simulink model "NCSEx3_sim"  (R2024b)
settings: Solver=VariableStepAuto  StartTime=0.0  StopTime=NCS.simTime  FixedStep=Td  RelTol=1e-3
InitFcn:
  | set_param(gcs, 'SimulationCommand', 'update')
values from neighbouring files (symbols this model uses):
  NCS = NcsStructureEx3(ncsPlant, 'simTime', simTime,                     'networkEffectsData', networkEffectsData,                     'controlParams', controlParams,                     'observerParams', observerParams)    [mainEx3.m]
undefined symbols (not defined in the file or in its folder): sfunchk
libraries: cstblocks x1, truetime x1
settings Model: Creator=jakob_ludwiger  LastModifiedBy=kala
settings SolverCC: AlgebraicLoopSolver=TrustRegion
settings DataIOCC: ReturnWorkspaceOutputs=off
settings DebuggingCC: UnconnectedInputMsg=warning  UnconnectedOutputMsg=warning  UnconnectedLineMsg=warning  ArithmeticOperatorsInVariantConditions=warning
settings ModelReferenceCC: EnableRefExpFcnMdlSchedulingChecks=on
settings SFSimCC: SimUseLocalCustomCode=off  CustomCodeUndefinedFunction=UseInterfaceOnly
settings RTWCC: RTWUseLocalCustomCode=off  GPUComputeCapability=3.5  DLArmComputeVersion=19.05
settings CodeAppCC: StateflowObjectComments=on

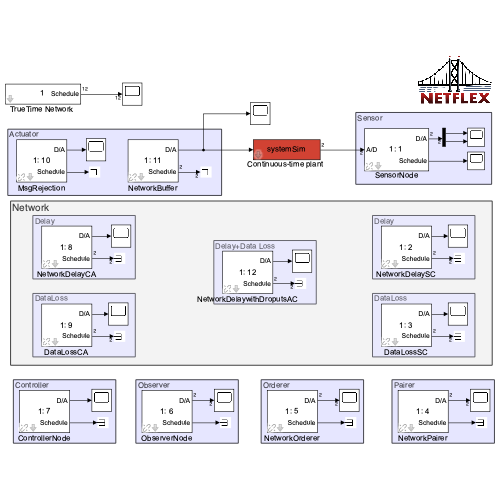
[thumbnail: Simulink's stored preview of the top-level diagram]
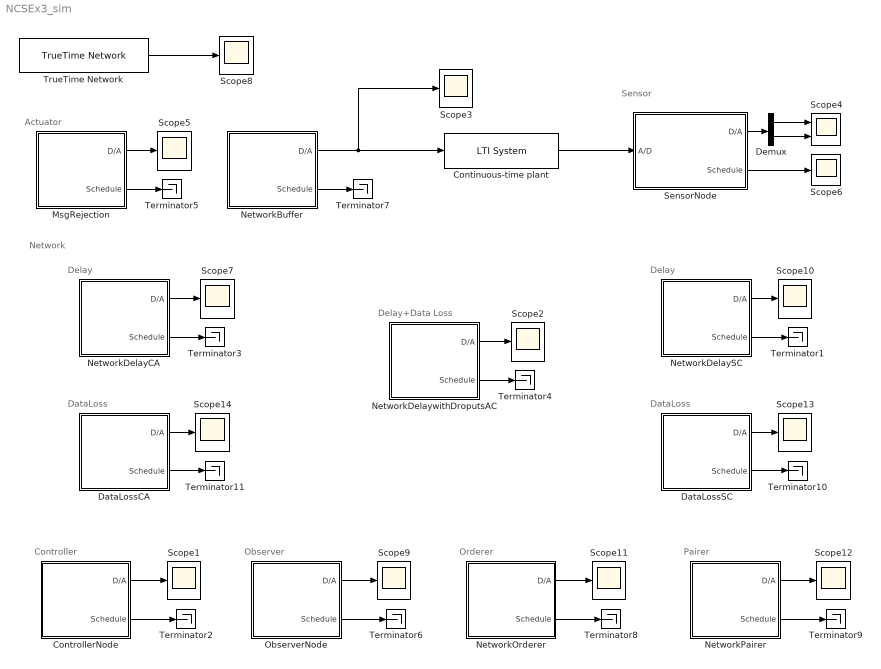
== system NCSEx3_sim ==
  note: Network
  note: Sensor
  note: Delay
  note: Delay
  note: Actuator
  note: Controller
  note: Delay+Data Loss
  note: Observer
  note: Orderer
  note: Pairer
  note: DataLoss
  note: DataLoss
  "Continuous-time plant " : cstblocks/LTI System  sys=systemSim  IC=initialState  PadeOrder=0
  ControllerNode : Subsystem  AncestorBlock=truetime/TrueTime Kernel  InitFcn=sfunchk(get_param(gcb,'sfun'));  mask{nodeObj=NCS.nodeMap('ControllerNode'), sfun=initFctWrapper, ntriggers=0, trigtype=falling, clockoffsetdrift=[0 0], schedoutput=on, battery=off, poweroutput=off, label=1: 7}
      mask prompts: nodeObj "Node Object"; sfun "Name of init function (MEX or MATLAB):"; ntriggers "Number of external triggers:"; trigtype "Trigger type:"; clockoffsetdrift "Local clock offset and drift:"; schedoutput "Show Schedule output port"; battery "Show Energy supply input port"; poweroutput "Show Power consumption output port"
      mask init:
      | set_param(gcb,'sfun', nodeObj.initFunctionWrapper)
      | %set_param(gcb,'args', [3 2])
      | args = nodeObj;
      | ninputsoutputs = [nodeObj.nIn nodeObj.nOut];
      | nwnodenbr = nodeObj.nodeNr;
      | ttkernel_callback(gcb,{sfun,args,ninputsoutputs,ntriggers,trigtype,nwnodenbr,clockoffsetdrift,schedoutput,battery,poweroutput})
      settings: ErrorFcn=ttkernel_error
      mask TypeOptions trigtype: rising | falling | either
      mask Display: disp(get_param(gcb,'label'))
  DataLossCA : Subsystem  AncestorBlock=truetime/TrueTime Kernel  InitFcn=sfunchk(get_param(gcb,'sfun'));  mask{nodeObj=NCS.nodeMap('NetworkDropoutCA'), sfun=initFctWrapper, ntriggers=0, trigtype=falling, clockoffsetdrift=[0 0], schedoutput=on, battery=off, poweroutput=off, label=1: 9}
      mask prompts: nodeObj "Node Object"; sfun "Name of init function (MEX or MATLAB):"; ntriggers "Number of external triggers:"; trigtype "Trigger type:"; clockoffsetdrift "Local clock offset and drift:"; schedoutput "Show Schedule output port"; battery "Show Energy supply input port"; poweroutput "Show Power consumption output port"
      mask init: same as NCSEx3_sim/ControllerNode
      settings: ErrorFcn=ttkernel_error
      mask TypeOptions trigtype: rising | falling | either
      mask Display: disp(get_param(gcb,'label'))
  DataLossSC : Subsystem  AncestorBlock=truetime/TrueTime Kernel  InitFcn=sfunchk(get_param(gcb,'sfun'));  mask{nodeObj=NCS.nodeMap('NetworkDropoutSC'), sfun=initFctWrapper, ntriggers=0, trigtype=falling, clockoffsetdrift=[0 0], schedoutput=on, battery=off, poweroutput=off, label=1: 3}
      mask prompts: nodeObj "Node Object"; sfun "Name of init function (MEX or MATLAB):"; ntriggers "Number of external triggers:"; trigtype "Trigger type:"; clockoffsetdrift "Local clock offset and drift:"; schedoutput "Show Schedule output port"; battery "Show Energy supply input port"; poweroutput "Show Power consumption output port"
      mask init: same as NCSEx3_sim/ControllerNode
      settings: ErrorFcn=ttkernel_error
      mask TypeOptions trigtype: rising | falling | either
      mask Display: disp(get_param(gcb,'label'))
  Demux : Demux  Outputs=2
  MsgRejection : Subsystem  AncestorBlock=truetime/TrueTime Kernel  InitFcn=sfunchk(get_param(gcb,'sfun'));  mask{nodeObj=NCS.nodeMap('MsgRejection'), sfun=initFctWrapper, ntriggers=0, trigtype=falling, clockoffsetdrift=[0 0], schedoutput=on, battery=off, poweroutput=off, label=1: 10}
      mask prompts: nodeObj "Node Object"; sfun "Name of init function (MEX or MATLAB):"; ntriggers "Number of external triggers:"; trigtype "Trigger type:"; clockoffsetdrift "Local clock offset and drift:"; schedoutput "Show Schedule output port"; battery "Show Energy supply input port"; poweroutput "Show Power consumption output port"
      mask init: same as NCSEx3_sim/ControllerNode
      settings: ErrorFcn=ttkernel_error
      mask TypeOptions trigtype: rising | falling | either
      mask Display: disp(get_param(gcb,'label'))
  NetworkBuffer : Subsystem  AncestorBlock=truetime/TrueTime Kernel  InitFcn=sfunchk(get_param(gcb,'sfun'));  mask{nodeObj=NCS.nodeMap('NetworkBuffer'), sfun=initFctWrapper, ntriggers=0, trigtype=falling, clockoffsetdrift=[0 0], schedoutput=on, battery=off, poweroutput=off, label=1: 11}
      mask prompts: nodeObj "Node Object"; sfun "Name of init function (MEX or MATLAB):"; ntriggers "Number of external triggers:"; trigtype "Trigger type:"; clockoffsetdrift "Local clock offset and drift:"; schedoutput "Show Schedule output port"; battery "Show Energy supply input port"; poweroutput "Show Power consumption output port"
      mask init: same as NCSEx3_sim/ControllerNode
      settings: ErrorFcn=ttkernel_error
      mask TypeOptions trigtype: rising | falling | either
      mask Display: disp(get_param(gcb,'label'))
  NetworkDelayCA : Subsystem  AncestorBlock=truetime/TrueTime Kernel  InitFcn=sfunchk(get_param(gcb,'sfun'));  mask{nodeObj=NCS.nodeMap('NetworkDelayCA'), sfun=initFctWrapper, ntriggers=0, trigtype=falling, clockoffsetdrift=[0 0], schedoutput=on, battery=off, poweroutput=off, label=1: 8}
      mask prompts: nodeObj "Node Object"; sfun "Name of init function (MEX or MATLAB):"; ntriggers "Number of external triggers:"; trigtype "Trigger type:"; clockoffsetdrift "Local clock offset and drift:"; schedoutput "Show Schedule output port"; battery "Show Energy supply input port"; poweroutput "Show Power consumption output port"
      mask init: same as NCSEx3_sim/ControllerNode
      settings: ErrorFcn=ttkernel_error
      mask TypeOptions trigtype: rising | falling | either
      mask Display: disp(get_param(gcb,'label'))
  NetworkDelaySC : Subsystem  AncestorBlock=truetime/TrueTime Kernel  InitFcn=sfunchk(get_param(gcb,'sfun'));  mask{nodeObj=NCS.nodeMap('NetworkDelaySC'), sfun=initFctWrapper, ntriggers=0, trigtype=falling, clockoffsetdrift=[0 0], schedoutput=on, battery=off, poweroutput=off, label=1: 2}
      mask prompts: nodeObj "Node Object"; sfun "Name of init function (MEX or MATLAB):"; ntriggers "Number of external triggers:"; trigtype "Trigger type:"; clockoffsetdrift "Local clock offset and drift:"; schedoutput "Show Schedule output port"; battery "Show Energy supply input port"; poweroutput "Show Power consumption output port"
      mask init: same as NCSEx3_sim/ControllerNode
      settings: ErrorFcn=ttkernel_error
      mask TypeOptions trigtype: rising | falling | either
      mask Display: disp(get_param(gcb,'label'))
  NetworkDelaywithDroputsAC : Subsystem  AncestorBlock=truetime/TrueTime Kernel  InitFcn=sfunchk(get_param(gcb,'sfun'));  mask{nodeObj=NCS.nodeMap('NetworkDelayWithDropoutsAC'), sfun=initFctWrapper, ntriggers=0, trigtype=falling, clockoffsetdrift=[0 0], schedoutput=on, battery=off, poweroutput=off, label=1: 12}
      mask prompts: nodeObj "Node Object"; sfun "Name of init function (MEX or MATLAB):"; ntriggers "Number of external triggers:"; trigtype "Trigger type:"; clockoffsetdrift "Local clock offset and drift:"; schedoutput "Show Schedule output port"; battery "Show Energy supply input port"; poweroutput "Show Power consumption output port"
      mask init: same as NCSEx3_sim/ControllerNode
      settings: ErrorFcn=ttkernel_error
      mask TypeOptions trigtype: rising | falling | either
      mask Display: disp(get_param(gcb,'label'))
  NetworkOrderer : Subsystem  AncestorBlock=truetime/TrueTime Kernel  InitFcn=sfunchk(get_param(gcb,'sfun'));  mask{nodeObj=NCS.nodeMap('NetworkOrderer'), sfun=initFctWrapper, ntriggers=0, trigtype=falling, clockoffsetdrift=[0 0], schedoutput=on, battery=off, poweroutput=off, label=1: 5}
      mask prompts: nodeObj "Node Object"; sfun "Name of init function (MEX or MATLAB):"; ntriggers "Number of external triggers:"; trigtype "Trigger type:"; clockoffsetdrift "Local clock offset and drift:"; schedoutput "Show Schedule output port"; battery "Show Energy supply input port"; poweroutput "Show Power consumption output port"
      mask init: same as NCSEx3_sim/ControllerNode
      settings: ErrorFcn=ttkernel_error
      mask TypeOptions trigtype: rising | falling | either
      mask Display: disp(get_param(gcb,'label'))
  NetworkPairer : Subsystem  AncestorBlock=truetime/TrueTime Kernel  InitFcn=sfunchk(get_param(gcb,'sfun'));  mask{nodeObj=NCS.nodeMap('NetworkPairer'), sfun=initFctWrapper, ntriggers=0, trigtype=falling, clockoffsetdrift=[0 0], schedoutput=on, battery=off, poweroutput=off, label=1: 4}
      mask prompts: nodeObj "Node Object"; sfun "Name of init function (MEX or MATLAB):"; ntriggers "Number of external triggers:"; trigtype "Trigger type:"; clockoffsetdrift "Local clock offset and drift:"; schedoutput "Show Schedule output port"; battery "Show Energy supply input port"; poweroutput "Show Power consumption output port"
      mask init: same as NCSEx3_sim/ControllerNode
      settings: ErrorFcn=ttkernel_error
      mask TypeOptions trigtype: rising | falling | either
      mask Display: disp(get_param(gcb,'label'))
  ObserverNode : Subsystem  AncestorBlock=truetime/TrueTime Kernel  InitFcn=sfunchk(get_param(gcb,'sfun'));  mask{nodeObj=NCS.nodeMap('ObserverNode'), sfun=initFctWrapper, ntriggers=0, trigtype=falling, clockoffsetdrift=[0 0], schedoutput=on, battery=off, poweroutput=off, label=1: 6}
      mask prompts: nodeObj "Node Object"; sfun "Name of init function (MEX or MATLAB):"; ntriggers "Number of external triggers:"; trigtype "Trigger type:"; clockoffsetdrift "Local clock offset and drift:"; schedoutput "Show Schedule output port"; battery "Show Energy supply input port"; poweroutput "Show Power consumption output port"
      mask init: same as NCSEx3_sim/ControllerNode
      settings: ErrorFcn=ttkernel_error
      mask TypeOptions trigtype: rising | falling | either
      mask Display: disp(get_param(gcb,'label'))
  Scope{1..3,5..14} (13 alike) : Scope
  Scope4 : Scope  NumInputPorts=2
  SensorNode : Subsystem  AncestorBlock=truetime/TrueTime Kernel  InitFcn=sfunchk(get_param(gcb,'sfun'));  mask{nodeObj=NCS.nodeMap('SensorNode'), sfun=initFctWrapper, ntriggers=0, trigtype=falling, clockoffsetdrift=[0 0], schedoutput=on, battery=off, poweroutput=off, label=1: 1}
      mask prompts: nodeObj "Node Object"; sfun "Name of init function (MEX or MATLAB):"; ntriggers "Number of external triggers:"; trigtype "Trigger type:"; clockoffsetdrift "Local clock offset and drift:"; schedoutput "Show Schedule output port"; battery "Show Energy supply input port"; poweroutput "Show Power consumption output port"
      mask init: same as NCSEx3_sim/ControllerNode
      settings: ErrorFcn=ttkernel_error
      mask TypeOptions trigtype: rising | falling | either
      mask Display: disp(get_param(gcb,'label'))
  Terminator{1..11} (11 alike) : Terminator
  "TrueTime Network " : truetime/TrueTime Network  nwtype=CSMA/CD (Ethernet)  nwnbr=1  nnodes=NCS.getMaxNodeNr  rate=1e8  minsize=200  lossprob=0  seed=0  bandwidths=[0.5 0.5]  slotsize=512  schedule=[1 1 2]  memsize=80000  buftype=Common buffer  overflow=Retransmit  dynSchedule=0  miniSlotSize=0  NIT=0  QSortMode=FIFO  sync=0  irtSchedule=0  nrtLength=0  nodeGraph=0  scheduleoutput=on
  wires:
  SensorNode/2(Schedule) -> Scope6/1
  SensorNode/1(D/A) -> Demux/1
  "Continuous-time plant "/1 -> SensorNode/1(A/D)
  "TrueTime Network "/1 -> Scope8/1
  NetworkDelaySC/2(Schedule) -> Terminator1/1
  NetworkDelaySC/1(D/A) -> Scope10/1
  NetworkDelayCA/1(D/A) -> Scope7/1
  NetworkDelayCA/2(Schedule) -> Terminator3/1
  MsgRejection/2(Schedule) -> Terminator5/1
  MsgRejection/1(D/A) -> Scope5/1
  NetworkBuffer/2(Schedule) -> Terminator7/1
  ControllerNode/1(D/A) -> Scope1/1
  ControllerNode/2(Schedule) -> Terminator2/1
  NetworkBuffer/1(D/A) -> Scope3/1, "Continuous-time plant "/1
  NetworkDelaywithDroputsAC/2(Schedule) -> Terminator4/1
  NetworkDelaywithDroputsAC/1(D/A) -> Scope2/1
  ObserverNode/2(Schedule) -> Terminator6/1
  ObserverNode/1(D/A) -> Scope9/1
  NetworkOrderer/1(D/A) -> Scope11/1
  NetworkOrderer/2(Schedule) -> Terminator8/1
  NetworkPairer/2(Schedule) -> Terminator9/1
  NetworkPairer/1(D/A) -> Scope12/1
  Demux/1 -> Scope4/1
  Demux/2 -> Scope4/2
  DataLossSC/1(D/A) -> Scope13/1
  DataLossSC/2(Schedule) -> Terminator10/1
  DataLossCA/2(Schedule) -> Terminator11/1
  DataLossCA/1(D/A) -> Scope14/1

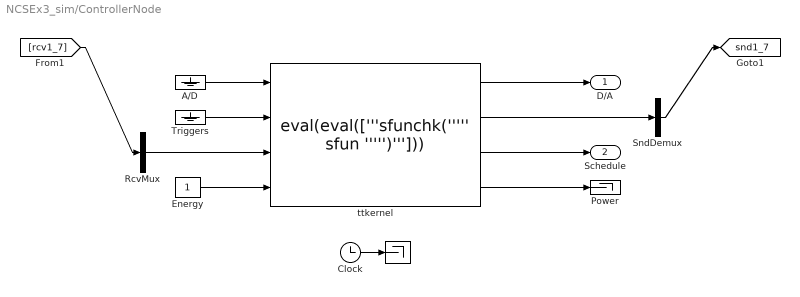
== system NCSEx3_sim/ControllerNode ==
  " " : Terminator
  A/D : Ground
  Clock : Clock
  Energy : Constant
  Power : Terminator
  RcvMux : Mux  Inputs=1
  SndDemux : Demux  Outputs=1
      settings: DisplayOption=none
  Triggers : Ground
  ttkernel : S-Function  FunctionName=eval(eval(['''sfunchk(''''' sfun ''''')''']))  Parameters=sfun, args, ninputsoutputs, ntriggers, trigtype, nwnodenbr, clockoffsetdrift  SFunctionDeploymentMode=off  EnableBusSupport=off
  D/A : Outport
  Schedule : Outport  Port=2
  tag scope: snd1_7=global
  wires:
  ttkernel/4 -> Power/1
  Energy/1 -> ttkernel/4
  A/D/1 -> ttkernel/1
  ttkernel/2 -> SndDemux/1
  ttkernel/1 -> D/A/1
  ttkernel/3 -> Schedule/1
  Triggers/1 -> ttkernel/2
  RcvMux/1 -> ttkernel/3
  Clock/1 -> " "/1
  [rcv1_7] -> RcvMux/1
  SndDemux/1 -> [snd1_7]

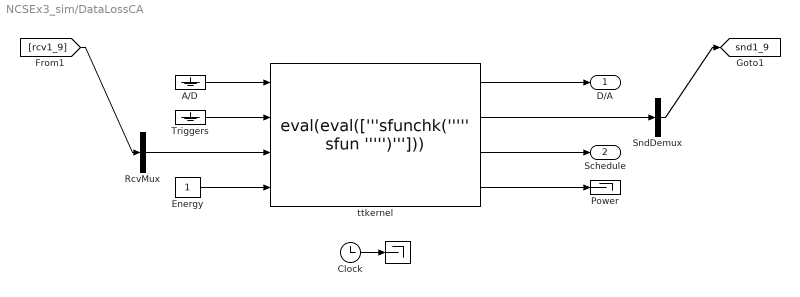
== system NCSEx3_sim/DataLossCA ==
  " " : Terminator
  A/D : Ground
  Clock : Clock
  Energy : Constant
  Power : Terminator
  RcvMux : Mux  Inputs=1
  SndDemux : Demux  Outputs=1
      settings: DisplayOption=none
  Triggers : Ground
  ttkernel : S-Function  FunctionName=eval(eval(['''sfunchk(''''' sfun ''''')''']))  Parameters=sfun, args, ninputsoutputs, ntriggers, trigtype, nwnodenbr, clockoffsetdrift  SFunctionDeploymentMode=off  EnableBusSupport=off
  D/A : Outport
  Schedule : Outport  Port=2
  tag scope: snd1_9=global
  wires:
  Clock/1 -> " "/1
  RcvMux/1 -> ttkernel/3
  Triggers/1 -> ttkernel/2
  ttkernel/3 -> Schedule/1
  ttkernel/1 -> D/A/1
  ttkernel/2 -> SndDemux/1
  A/D/1 -> ttkernel/1
  Energy/1 -> ttkernel/4
  ttkernel/4 -> Power/1
  [rcv1_9] -> RcvMux/1
  SndDemux/1 -> [snd1_9]

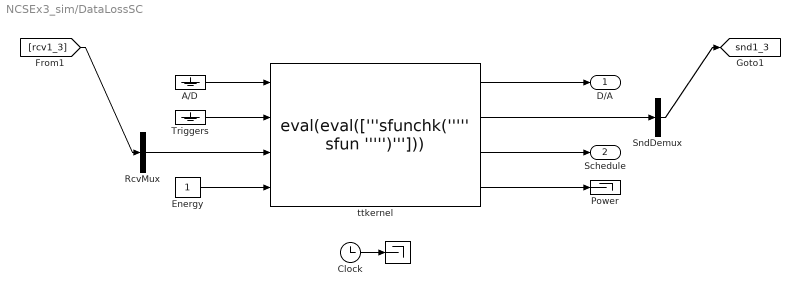
== system NCSEx3_sim/DataLossSC ==
  " " : Terminator
  A/D : Ground
  Clock : Clock
  Energy : Constant
  Power : Terminator
  RcvMux : Mux  Inputs=1
  SndDemux : Demux  Outputs=1
      settings: DisplayOption=none
  Triggers : Ground
  ttkernel : S-Function  FunctionName=eval(eval(['''sfunchk(''''' sfun ''''')''']))  Parameters=sfun, args, ninputsoutputs, ntriggers, trigtype, nwnodenbr, clockoffsetdrift  SFunctionDeploymentMode=off  EnableBusSupport=off
  D/A : Outport
  Schedule : Outport  Port=2
  tag scope: snd1_3=global
  wires:
  ttkernel/4 -> Power/1
  Energy/1 -> ttkernel/4
  A/D/1 -> ttkernel/1
  ttkernel/2 -> SndDemux/1
  ttkernel/1 -> D/A/1
  ttkernel/3 -> Schedule/1
  Triggers/1 -> ttkernel/2
  RcvMux/1 -> ttkernel/3
  Clock/1 -> " "/1
  [rcv1_3] -> RcvMux/1
  SndDemux/1 -> [snd1_3]

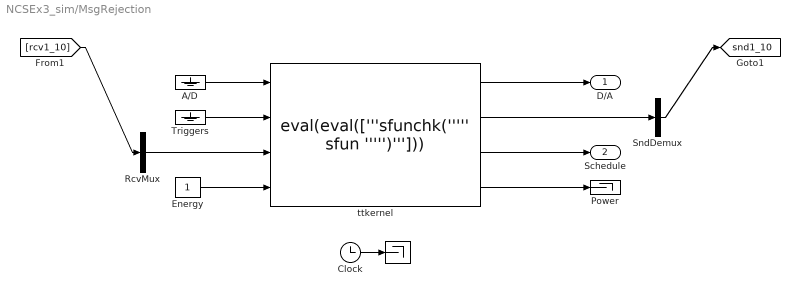
== system NCSEx3_sim/MsgRejection ==
  " " : Terminator
  A/D : Ground
  Clock : Clock
  Energy : Constant
  Power : Terminator
  RcvMux : Mux  Inputs=1
  SndDemux : Demux  Outputs=1
      settings: DisplayOption=none
  Triggers : Ground
  ttkernel : S-Function  FunctionName=eval(eval(['''sfunchk(''''' sfun ''''')''']))  Parameters=sfun, args, ninputsoutputs, ntriggers, trigtype, nwnodenbr, clockoffsetdrift  SFunctionDeploymentMode=off  EnableBusSupport=off
  D/A : Outport
  Schedule : Outport  Port=2
  tag scope: snd1_10=global
  wires:
  Clock/1 -> " "/1
  RcvMux/1 -> ttkernel/3
  Triggers/1 -> ttkernel/2
  ttkernel/3 -> Schedule/1
  ttkernel/1 -> D/A/1
  ttkernel/2 -> SndDemux/1
  A/D/1 -> ttkernel/1
  Energy/1 -> ttkernel/4
  ttkernel/4 -> Power/1
  [rcv1_10] -> RcvMux/1
  SndDemux/1 -> [snd1_10]

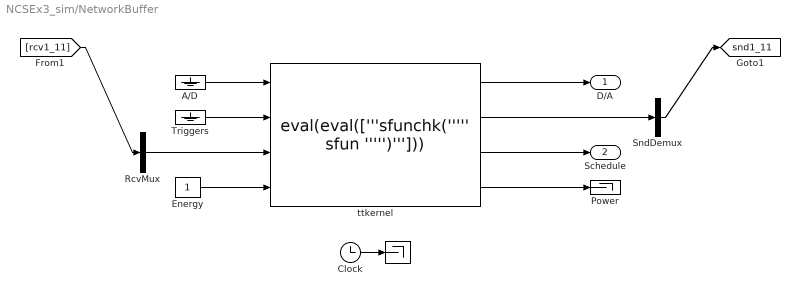
== system NCSEx3_sim/NetworkBuffer ==
  " " : Terminator
  A/D : Ground
  Clock : Clock
  Energy : Constant
  Power : Terminator
  RcvMux : Mux  Inputs=1
  SndDemux : Demux  Outputs=1
      settings: DisplayOption=none
  Triggers : Ground
  ttkernel : S-Function  FunctionName=eval(eval(['''sfunchk(''''' sfun ''''')''']))  Parameters=sfun, args, ninputsoutputs, ntriggers, trigtype, nwnodenbr, clockoffsetdrift  SFunctionDeploymentMode=off  EnableBusSupport=off
  D/A : Outport
  Schedule : Outport  Port=2
  tag scope: snd1_11=global
  wires:
  ttkernel/4 -> Power/1
  Energy/1 -> ttkernel/4
  A/D/1 -> ttkernel/1
  ttkernel/2 -> SndDemux/1
  ttkernel/1 -> D/A/1
  ttkernel/3 -> Schedule/1
  Triggers/1 -> ttkernel/2
  RcvMux/1 -> ttkernel/3
  Clock/1 -> " "/1
  [rcv1_11] -> RcvMux/1
  SndDemux/1 -> [snd1_11]

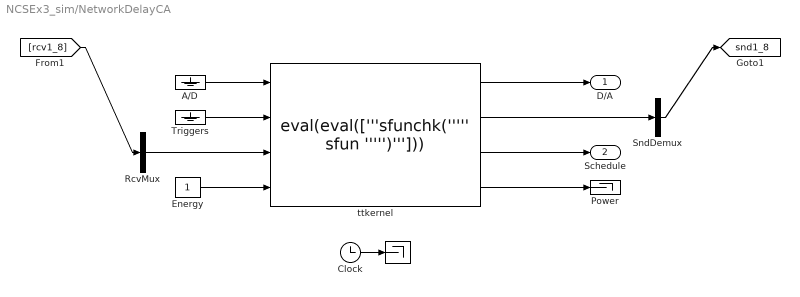
== system NCSEx3_sim/NetworkDelayCA ==
  " " : Terminator
  A/D : Ground
  Clock : Clock
  Energy : Constant
  Power : Terminator
  RcvMux : Mux  Inputs=1
  SndDemux : Demux  Outputs=1
      settings: DisplayOption=none
  Triggers : Ground
  ttkernel : S-Function  FunctionName=eval(eval(['''sfunchk(''''' sfun ''''')''']))  Parameters=sfun, args, ninputsoutputs, ntriggers, trigtype, nwnodenbr, clockoffsetdrift  SFunctionDeploymentMode=off  EnableBusSupport=off
  D/A : Outport
  Schedule : Outport  Port=2
  tag scope: snd1_8=global
  wires:
  ttkernel/4 -> Power/1
  Energy/1 -> ttkernel/4
  A/D/1 -> ttkernel/1
  ttkernel/2 -> SndDemux/1
  ttkernel/1 -> D/A/1
  ttkernel/3 -> Schedule/1
  Triggers/1 -> ttkernel/2
  RcvMux/1 -> ttkernel/3
  Clock/1 -> " "/1
  [rcv1_8] -> RcvMux/1
  SndDemux/1 -> [snd1_8]

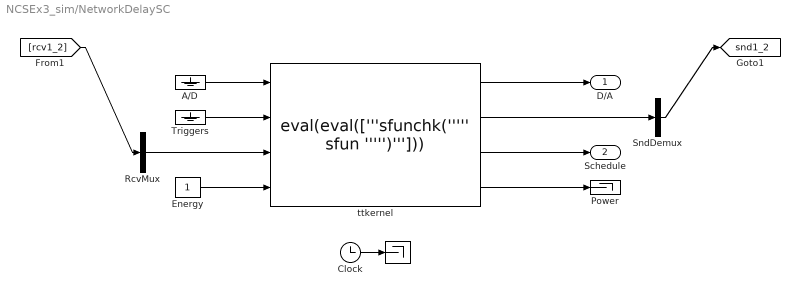
== system NCSEx3_sim/NetworkDelaySC ==
  " " : Terminator
  A/D : Ground
  Clock : Clock
  Energy : Constant
  Power : Terminator
  RcvMux : Mux  Inputs=1
  SndDemux : Demux  Outputs=1
      settings: DisplayOption=none
  Triggers : Ground
  ttkernel : S-Function  FunctionName=eval(eval(['''sfunchk(''''' sfun ''''')''']))  Parameters=sfun, args, ninputsoutputs, ntriggers, trigtype, nwnodenbr, clockoffsetdrift  SFunctionDeploymentMode=off  EnableBusSupport=off
  D/A : Outport
  Schedule : Outport  Port=2
  tag scope: snd1_2=global
  wires:
  Clock/1 -> " "/1
  RcvMux/1 -> ttkernel/3
  Triggers/1 -> ttkernel/2
  ttkernel/3 -> Schedule/1
  ttkernel/1 -> D/A/1
  ttkernel/2 -> SndDemux/1
  A/D/1 -> ttkernel/1
  Energy/1 -> ttkernel/4
  ttkernel/4 -> Power/1
  [rcv1_2] -> RcvMux/1
  SndDemux/1 -> [snd1_2]

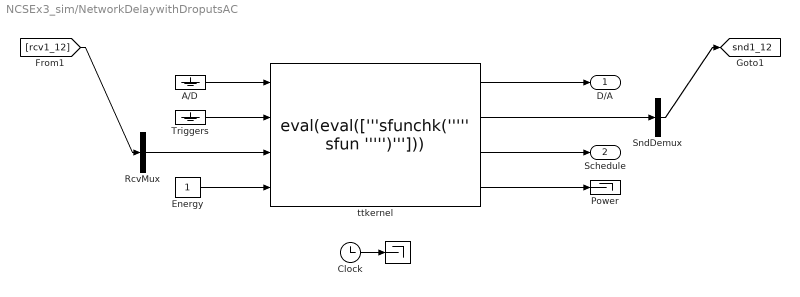
== system NCSEx3_sim/NetworkDelaywithDroputsAC ==
  " " : Terminator
  A/D : Ground
  Clock : Clock
  Energy : Constant
  Power : Terminator
  RcvMux : Mux  Inputs=1
  SndDemux : Demux  Outputs=1
      settings: DisplayOption=none
  Triggers : Ground
  ttkernel : S-Function  FunctionName=eval(eval(['''sfunchk(''''' sfun ''''')''']))  Parameters=sfun, args, ninputsoutputs, ntriggers, trigtype, nwnodenbr, clockoffsetdrift  SFunctionDeploymentMode=off  EnableBusSupport=off
  D/A : Outport
  Schedule : Outport  Port=2
  tag scope: snd1_12=global
  wires:
  Clock/1 -> " "/1
  RcvMux/1 -> ttkernel/3
  Triggers/1 -> ttkernel/2
  ttkernel/3 -> Schedule/1
  ttkernel/1 -> D/A/1
  ttkernel/2 -> SndDemux/1
  A/D/1 -> ttkernel/1
  Energy/1 -> ttkernel/4
  ttkernel/4 -> Power/1
  [rcv1_12] -> RcvMux/1
  SndDemux/1 -> [snd1_12]

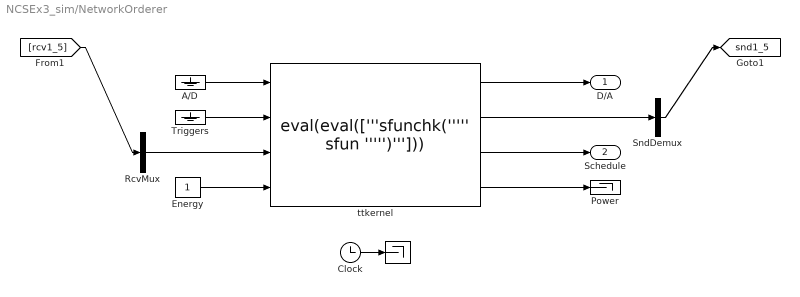
== system NCSEx3_sim/NetworkOrderer ==
  " " : Terminator
  A/D : Ground
  Clock : Clock
  Energy : Constant
  Power : Terminator
  RcvMux : Mux  Inputs=1
  SndDemux : Demux  Outputs=1
      settings: DisplayOption=none
  Triggers : Ground
  ttkernel : S-Function  FunctionName=eval(eval(['''sfunchk(''''' sfun ''''')''']))  Parameters=sfun, args, ninputsoutputs, ntriggers, trigtype, nwnodenbr, clockoffsetdrift  SFunctionDeploymentMode=off  EnableBusSupport=off
  D/A : Outport
  Schedule : Outport  Port=2
  tag scope: snd1_5=global
  wires:
  ttkernel/4 -> Power/1
  Energy/1 -> ttkernel/4
  A/D/1 -> ttkernel/1
  ttkernel/2 -> SndDemux/1
  ttkernel/1 -> D/A/1
  ttkernel/3 -> Schedule/1
  Triggers/1 -> ttkernel/2
  RcvMux/1 -> ttkernel/3
  Clock/1 -> " "/1
  [rcv1_5] -> RcvMux/1
  SndDemux/1 -> [snd1_5]

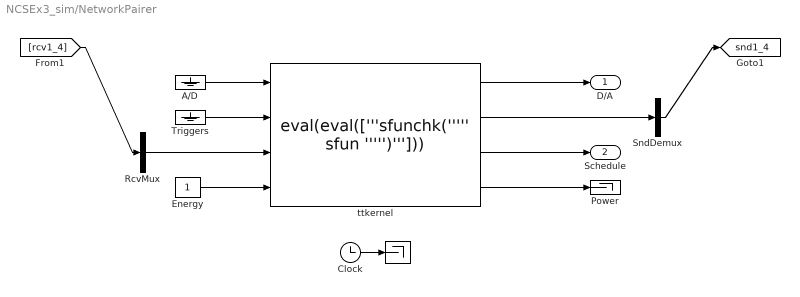
== system NCSEx3_sim/NetworkPairer ==
  " " : Terminator
  A/D : Ground
  Clock : Clock
  Energy : Constant
  Power : Terminator
  RcvMux : Mux  Inputs=1
  SndDemux : Demux  Outputs=1
      settings: DisplayOption=none
  Triggers : Ground
  ttkernel : S-Function  FunctionName=eval(eval(['''sfunchk(''''' sfun ''''')''']))  Parameters=sfun, args, ninputsoutputs, ntriggers, trigtype, nwnodenbr, clockoffsetdrift  SFunctionDeploymentMode=off  EnableBusSupport=off
  D/A : Outport
  Schedule : Outport  Port=2
  tag scope: snd1_4=global
  wires:
  Clock/1 -> " "/1
  RcvMux/1 -> ttkernel/3
  Triggers/1 -> ttkernel/2
  ttkernel/3 -> Schedule/1
  ttkernel/1 -> D/A/1
  ttkernel/2 -> SndDemux/1
  A/D/1 -> ttkernel/1
  Energy/1 -> ttkernel/4
  ttkernel/4 -> Power/1
  [rcv1_4] -> RcvMux/1
  SndDemux/1 -> [snd1_4]

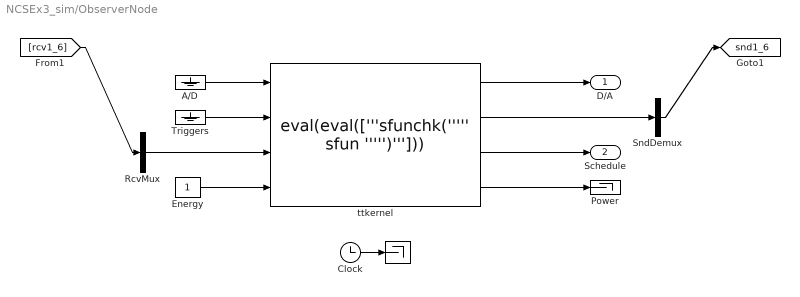
== system NCSEx3_sim/ObserverNode ==
  " " : Terminator
  A/D : Ground
  Clock : Clock
  Energy : Constant
  Power : Terminator
  RcvMux : Mux  Inputs=1
  SndDemux : Demux  Outputs=1
      settings: DisplayOption=none
  Triggers : Ground
  ttkernel : S-Function  FunctionName=eval(eval(['''sfunchk(''''' sfun ''''')''']))  Parameters=sfun, args, ninputsoutputs, ntriggers, trigtype, nwnodenbr, clockoffsetdrift  SFunctionDeploymentMode=off  EnableBusSupport=off
  D/A : Outport
  Schedule : Outport  Port=2
  tag scope: snd1_6=global
  wires:
  Clock/1 -> " "/1
  RcvMux/1 -> ttkernel/3
  Triggers/1 -> ttkernel/2
  ttkernel/3 -> Schedule/1
  ttkernel/1 -> D/A/1
  ttkernel/2 -> SndDemux/1
  A/D/1 -> ttkernel/1
  Energy/1 -> ttkernel/4
  ttkernel/4 -> Power/1
  [rcv1_6] -> RcvMux/1
  SndDemux/1 -> [snd1_6]

== system NCSEx3_sim/SensorNode ==
  A/D : Inport
  " " : Terminator
  Clock : Clock
  Energy : Constant
  Power : Terminator
  RcvMux : Mux  Inputs=1
  SndDemux : Demux  Outputs=1
      settings: DisplayOption=none
  Triggers : Ground
  ttkernel : S-Function  FunctionName=eval(eval(['''sfunchk(''''' sfun ''''')''']))  Parameters=sfun, args, ninputsoutputs, ntriggers, trigtype, nwnodenbr, clockoffsetdrift  SFunctionDeploymentMode=off  EnableBusSupport=off
  D/A : Outport
  Schedule : Outport  Port=2
  tag scope: snd1_1=global
  wires:
  ttkernel/4 -> Power/1
  Energy/1 -> ttkernel/4
  A/D/1 -> ttkernel/1
  ttkernel/2 -> SndDemux/1
  ttkernel/1 -> D/A/1
  ttkernel/3 -> Schedule/1
  Triggers/1 -> ttkernel/2
  RcvMux/1 -> ttkernel/3
  Clock/1 -> " "/1
  [rcv1_1] -> RcvMux/1
  SndDemux/1 -> [snd1_1]
